simulink model "kamerol"  (R2021b)
settings: Solver=VariableStepAuto  StartTime=0.0  StopTime=10.0  RelTol=1e-3
undefined symbols (not defined in the file): admireDB
libraries: simulink_extras x104, simulink x24, sharedutil x1
(part 3 of 14)

== system kamerol/Aerodynamics/CentripetalForceCoefficient/MachRegion4/Ccday ==
  in_bus : Inport
  Bus Selector : BusSelector  OutputSignals=AeroIn_Bus.angleOfAttack_deg,AeroIn_Bus.dEY,AeroIn_Bus.mach_nd,AeroIn_Bus.qacorr,eoeff,AeroIn_Bus.dAY
  Ccday_ : Subsystem
  Ccday : Outport
  wires:
  Bus Selector/6 -> Ccday_/6(dAY)  "<dAY>"
  Bus Selector/5 -> Ccday_/5(eoeff)  "<eoeff>"
  Bus Selector/4 -> Ccday_/4(qacorr)  "<qacorr>"
  Bus Selector/3 -> Ccday_/3(mach_nd)  "<mach_nd>"
  Bus Selector/2 -> Ccday_/2(dEY)  "<dEY>"
  Bus Selector/1 -> Ccday_/1(angleOfAttack_deg)  "<angleOfAttack_deg>"
  Ccday_/1(Ccday) -> Ccday/1
  in_bus/1 -> Bus Selector/1  "in_bus"

== system kamerol/Aerodynamics/CentripetalForceCoefficient/MachRegion4/Ccdayb ==
  Constant : Constant  Value=0
  Ccdayb : Outport
  wires:
  Constant/1 -> Ccdayb/1

== system kamerol/Aerodynamics/CentripetalForceCoefficient/MachRegion4/Ccdna ==
  in_bus : Inport
  Bus Selector : BusSelector  OutputSignals=AeroIn_Bus.angleOfAttack_deg,AeroIn_Bus.mach_nd,AeroIn_Bus.dNA
  Ccdna_ : Subsystem
  Ccdna : Outport
  wires:
  Bus Selector/1 -> Ccdna_/1(angleOfAttack_deg)  "<angleOfAttack_deg>"
  Bus Selector/3 -> Ccdna_/3(dNA)  "<dNA>"
  Bus Selector/2 -> Ccdna_/2(mach_nd)  "<mach_nd>"
  in_bus/1 -> Bus Selector/1  "in_bus"
  Ccdna_/1(Ccdna) -> Ccdna/1

== system kamerol/Aerodynamics/CentripetalForceCoefficient/MachRegion4/Ccdr ==
  in_bus : Inport
  Bus Selector : BusSelector  OutputSignals=AeroIn_Bus.angleOfAttack_deg,AeroIn_Bus.mach_nd,AeroIn_Bus.rud_deg,AeroIn_Bus.qacorr
  Ccdr_ : Subsystem
  Ccdr : Outport
  wires:
  Bus Selector/1 -> Ccdr_/1(angleOfAttack_deg)  "<angleOfAttack_deg>"
  Bus Selector/2 -> Ccdr_/2(mach_nd)  "<mach_nd>"
  Bus Selector/3 -> Ccdr_/3(dR)  "<rud_deg>"
  Bus Selector/4 -> Ccdr_/4(qacorr)  "<qacorr>"
  Ccdr_/1(Ccdr) -> Ccdr/1
  in_bus/1 -> Bus Selector/1  "in_bus"

== system kamerol/Aerodynamics/CentripetalForceCoefficient/MachRegion4/Ccp ==
  in_bus : Inport
  Bus Selector : BusSelector  OutputSignals=AeroIn_Bus.angleOfAttack_deg,AeroIn_Bus.mach_nd,AeroIn_Bus.pc
  Ccp_ : Subsystem
  Ccp : Outport
  wires:
  Bus Selector/1 -> Ccp_/1(angleOfAttack_deg)  "<angleOfAttack_deg>"
  Bus Selector/2 -> Ccp_/2(mach_nd)  "<mach_nd>"
  Bus Selector/3 -> Ccp_/3(pc)  "<pc>"
  in_bus/1 -> Bus Selector/1  "in_bus"
  Ccp_/1(Ccp) -> Ccp/1

== system kamerol/Aerodynamics/CentripetalForceCoefficient/MachRegion4/Ccpbeta ==
  Constant : Constant  Value=0
  Ccpbeta : Outport
  wires:
  Constant/1 -> Ccpbeta/1

== system kamerol/Aerodynamics/CentripetalForceCoefficient/MachRegion4/Ccr ==
  in_bus : Inport
  Bus Selector : BusSelector  OutputSignals=AeroIn_Bus.mach_nd,AeroIn_Bus.qacorr,AeroIn_Bus.rc
  Ccr_ : Subsystem
  Ccr : Outport
  wires:
  Bus Selector/3 -> Ccr_/3(rc)  "<rc>"
  Bus Selector/2 -> Ccr_/2(qacorr)  "<qacorr>"
  Bus Selector/1 -> Ccr_/1(mach_nd)  "<mach_nd>"
  in_bus/1 -> Bus Selector/1  "in_bus"
  Ccr_/1(Ccr) -> Ccr/1

== system kamerol/Aerodynamics/CentripetalForceCoefficient/MachRegion4/Ccrbeta ==
  Constant : Constant  Value=0
  Ccrbeta : Outport
  wires:
  Constant/1 -> Ccrbeta/1

== system kamerol/Aerodynamics/CentripetalForceCoefficient/MachRegion4/eoeff ==
  AeroIn_Bus : Inport
  Bus Selector : BusSelector  OutputSignals=mach_nd
  CCDAYOD_M : Lookup_n-D  NumberOfTableDimensions=1  BreakpointsForDimension1=admireDB.aerodata_asym_ext.CCDAYOD.breakpoints.M  BreakpointsForDimension3=[5, 7]  Table=admireDB.aerodata_asym_ext.CCDAYOD.newTable  ExtrapMethod=Clip  InternalRulePriority=Speed  RndMeth=Simplest  InputSameDT=on
  Constant : Constant
  Sum : Sum  Inputs=-+|
  eoeff : Outport
  eieff : Outport  Port=2
  wires:
  Sum/1 -> eieff/1
  CCDAYOD_M/1 -> eoeff/1, Sum/1
  Constant/1 -> Sum/2
  Bus Selector/1 -> CCDAYOD_M/1  "<mach_nd>"
  AeroIn_Bus/1 -> Bus Selector/1

== system kamerol/Aerodynamics/NormalForceCoefficient/MachRegion1/Cnalfa ==
  in_bus : Inport
  Bus Selector : BusSelector  OutputSignals=AeroIn_Bus.angleOfAttack_deg,AeroIn_Bus.mach_nd,AeroIn_Bus.qacorr
  CNDEAL_DE_ALFA : Lookup_n-D  BreakpointsForDimension1=admireDB.aerodata_sym.CNDEAL.breakpoints.ALFA  BreakpointsForDimension2=admireDB.aerodata_sym.CNDEAL.breakpoints.DE  BreakpointsForDimension3=[5, 7]  Table=admireDB.aerodata_sym.CNDEAL.newTable  ExtrapMethod=Clip  InternalRulePriority=Speed  RndMeth=Simplest  InputSameDT=on
      settings: InputPortMap=u0,u1
  CNEA_QA_M : Lookup_n-D  BreakpointsForDimension1=admireDB.aerodata_sym.CNEA.breakpoints.M  BreakpointsForDimension2=admireDB.aerodata_sym.CNEA.breakpoints.QA  BreakpointsForDimension3=[5, 7]  Table=admireDB.aerodata_sym.CNEA.newTable  ExtrapMethod=Clip  InternalRulePriority=Speed  RndMeth=Simplest  InputSameDT=on
      settings: InputPortMap=u0,u1
  Constant : Constant  Value=0
  Product : Product
  Cnalfa : Outport
  wires:
  Product/1 -> Cnalfa/1
  CNDEAL_DE_ALFA/1 -> Product/1
  CNEA_QA_M/1 -> Product/2
  Bus Selector/2 -> CNEA_QA_M/1  "<mach_nd>"
  Bus Selector/3 -> CNEA_QA_M/2  "<qacorr>"
  Constant/1 -> CNDEAL_DE_ALFA/2
  Bus Selector/1 -> CNDEAL_DE_ALFA/1  "<angleOfAttack_deg>"
  in_bus/1 -> Bus Selector/1  "in_bus"

== system kamerol/Aerodynamics/NormalForceCoefficient/MachRegion1/Cnalfad ==
  in_bus : Inport
  Abs : Abs
  Bus Selector : BusSelector  OutputSignals=AeroIn_Bus.mach_nd,AeroIn_Bus.angleOfAttack_deg,AeroIn_Bus.alfad
  CNADAM_ALFA_M : Lookup_n-D  BreakpointsForDimension1=admireDB.aerodata_sym.CNADAM.breakpoints.M  BreakpointsForDimension2=admireDB.aerodata_sym.CNADAM.breakpoints.ALFA  BreakpointsForDimension3=[5, 7]  Table=admireDB.aerodata_sym.CNADAM.newTable  ExtrapMethod=Clip  InternalRulePriority=Speed  RndMeth=Simplest  InputSameDT=on
      settings: InputPortMap=u0,u1
  Product : Product
  Cnalfad : Outport
  wires:
  Abs/1 -> CNADAM_ALFA_M/2
  Bus Selector/1 -> CNADAM_ALFA_M/1  "<mach_nd>"
  Product/1 -> Cnalfad/1
  in_bus/1 -> Bus Selector/1  "in_bus"
  Bus Selector/2 -> Abs/1  "<angleOfAttack_deg>"
  CNADAM_ALFA_M/1 -> Product/1
  Bus Selector/3 -> Product/2  "<alfad>"

== system kamerol/Aerodynamics/NormalForceCoefficient/MachRegion1/Cnbasic ==
  in_bus : Inport
  Bus Selector : BusSelector  OutputSignals=AeroIn_Bus.mach_nd,AeroIn_Bus.qacorr
  CNEZERO_QA_M : Lookup_n-D  BreakpointsForDimension1=admireDB.aerodata_sym.CNEZERO.breakpoints.M  BreakpointsForDimension2=admireDB.aerodata_sym.CNEZERO.breakpoints.QA  BreakpointsForDimension3=[5, 7]  Table=admireDB.aerodata_sym.CNEZERO.newTable  ExtrapMethod=Clip  InternalRulePriority=Speed  RndMeth=Simplest  InputSameDT=on
      settings: InputPortMap=u0,u1
  CNZERO_M : Lookup_n-D  NumberOfTableDimensions=1  BreakpointsForDimension1=admireDB.aerodata_sym.CNZERO.breakpoints.M  BreakpointsForDimension3=[5, 7]  Table=admireDB.aerodata_sym.CNZERO.newTable  ExtrapMethod=Clip  InternalRulePriority=Speed  RndMeth=Simplest  InputSameDT=on
  Sum1 : Sum  Inputs=|++
  Cnbasic : Outport
  wires:
  CNEZERO_QA_M/1 -> Sum1/2
  CNZERO_M/1 -> Sum1/1
  Bus Selector/2 -> CNEZERO_QA_M/2  "<qacorr>"
  Bus Selector/1 -> CNZERO_M/1, CNEZERO_QA_M/1  "<mach_nd>"
  Sum1/1 -> Cnbasic/1
  in_bus/1 -> Bus Selector/1  "in_bus"

== system kamerol/Aerodynamics/NormalForceCoefficient/MachRegion1/Cnbeta ==
  in_bus : Inport
  Abs : Abs
  Bus Selector : BusSelector  OutputSignals=AeroIn_Bus.angleOfAttack_deg,AeroIn_Bus.dN,AeroIn_Bus.angleOfSideslip_deg
  CNBETA_DN_ALFA : Lookup_n-D  BreakpointsForDimension1=admireDB.aerodata_sym.CNBETA.breakpoints.ALFA  BreakpointsForDimension2=admireDB.aerodata_sym.CNBETA.breakpoints.DN  BreakpointsForDimension3=[5, 7]  Table=admireDB.aerodata_sym.CNBETA.newTable  ExtrapMethod=Clip  InternalRulePriority=Speed  RndMeth=Simplest  InputSameDT=on
      settings: InputPortMap=u0,u1
  CNKB_BETA : Lookup_n-D  NumberOfTableDimensions=1  BreakpointsForDimension1=admireDB.aerodata_sym.CNKB.breakpoints.BETA  BreakpointsForDimension3=[5, 7]  Table=admireDB.aerodata_sym.CNKB.newTable  ExtrapMethod=Clip  InternalRulePriority=Speed  RndMeth=Simplest  InputSameDT=on
  Product : Product
  Cnbeta : Outport
  wires:
  Product/1 -> Cnbeta/1
  CNBETA_DN_ALFA/1 -> Product/1
  CNKB_BETA/1 -> Product/2
  Abs/1 -> CNKB_BETA/1
  Bus Selector/3 -> Abs/1  "<angleOfSideslip_deg>"
  in_bus/1 -> Bus Selector/1  "in_bus"
  Bus Selector/2 -> CNBETA_DN_ALFA/2  "<dN>"
  Bus Selector/1 -> CNBETA_DN_ALFA/1  "<angleOfAttack_deg>"

== system kamerol/Aerodynamics/NormalForceCoefficient/MachRegion1/Cncai ==
  in_bus : Inport
  Bus Selector : BusSelector  OutputSignals=AeroIn_Bus.angleOfAttack_deg,AeroIn_Bus.cai
  CNCAI_CAI_ALFA : Lookup_n-D  BreakpointsForDimension1=admireDB.aerodata_sym.CNCAI.breakpoints.ALFA  BreakpointsForDimension2=admireDB.aerodata_sym.CNCAI.breakpoints.CAI  BreakpointsForDimension3=[5, 7]  Table=admireDB.aerodata_sym.CNCAI.newTable  ExtrapMethod=Clip  InternalRulePriority=Speed  RndMeth=Simplest  InputSameDT=on
      settings: InputPortMap=u0,u1
  Cncai : Outport
  wires:
  Bus Selector/1 -> CNCAI_CAI_ALFA/1  "<angleOfAttack_deg>"
  Bus Selector/2 -> CNCAI_CAI_ALFA/2  "<cai>"
  in_bus/1 -> Bus Selector/1  "in_bus"
  CNCAI_CAI_ALFA/1 -> Cncai/1

== system kamerol/Aerodynamics/NormalForceCoefficient/MachRegion1/Cndedn ==
  in_bus : Inport
  Bus Selector : BusSelector  OutputSignals=AeroIn_Bus.angleOfAttack_deg,AeroIn_Bus.dE,AeroIn_Bus.dN
  CNDNDE_ALFA_DE_DN : Lookup_n-D  NumberOfTableDimensions=3  BreakpointsForDimension1=admireDB.aerodata_sym.CNDNDE.breakpoints.ALFA  BreakpointsForDimension2=admireDB.aerodata_sym.CNDNDE.breakpoints.DE  BreakpointsForDimension3=admireDB.aerodata_sym.CNDNDE.breakpoints.DN  Table=admireDB.aerodata_sym.CNDNDE.newTable  ExtrapMethod=Clip  InternalRulePriority=Speed  RndMeth=Simplest  InputSameDT=on
      settings: InputPortMap=u0,u1,u2
  Cndedn : Outport
  wires:
  CNDNDE_ALFA_DE_DN/1 -> Cndedn/1
  Bus Selector/3 -> CNDNDE_ALFA_DE_DN/3  "<dN>"
  Bus Selector/2 -> CNDNDE_ALFA_DE_DN/2  "<dE>"
  Bus Selector/1 -> CNDNDE_ALFA_DE_DN/1  "<angleOfAttack_deg>"
  in_bus/1 -> Bus Selector/1  "in_bus"

== system kamerol/Aerodynamics/NormalForceCoefficient/MachRegion1/Cndei ==
  in_bus : Inport
  Bus Selector : BusSelector  OutputSignals=eieff,AeroIn_Bus.angleOfAttack_deg,AeroIn_Bus.dEI,AeroIn_Bus.mach_nd,AeroIn_Bus.qacorr
  CNDEAL_DE_ALFA : Lookup_n-D  BreakpointsForDimension1=admireDB.aerodata_sym.CNDEAL.breakpoints.ALFA  BreakpointsForDimension2=admireDB.aerodata_sym.CNDEAL.breakpoints.DE  BreakpointsForDimension3=[5, 7]  Table=admireDB.aerodata_sym.CNDEAL.newTable  ExtrapMethod=Clip  InternalRulePriority=Speed  RndMeth=Simplest  InputSameDT=on
      settings: InputPortMap=u0,u1
  CNDEAL_DE_ALFA1 : Lookup_n-D  BreakpointsForDimension1=admireDB.aerodata_sym.CNDEAL.breakpoints.ALFA  BreakpointsForDimension2=admireDB.aerodata_sym.CNDEAL.breakpoints.DE  BreakpointsForDimension3=[5, 7]  Table=admireDB.aerodata_sym.CNDEAL.newTable  ExtrapMethod=Clip  InternalRulePriority=Speed  RndMeth=Simplest  InputSameDT=on
      settings: InputPortMap=u0,u1
  CNEDEI_QA_M : Lookup_n-D  BreakpointsForDimension1=admireDB.aerodata_sym.CNEDEI.breakpoints.M  BreakpointsForDimension2=admireDB.aerodata_sym.CNEDEI.breakpoints.QA  BreakpointsForDimension3=[5, 7]  Table=admireDB.aerodata_sym.CNEDEI.newTable  ExtrapMethod=Clip  InternalRulePriority=Speed  RndMeth=Simplest  InputSameDT=on
      settings: InputPortMap=u0,u1
  Constant : Constant  Value=0
  Product : Product  Inputs=3
  Sum : Sum  Inputs=|+-
  Cndei : Outport
  wires:
  CNEDEI_QA_M/1 -> Product/3
  Sum/1 -> Product/2
  Bus Selector/1 -> Product/1  "<eieff>"
  Bus Selector/4 -> CNEDEI_QA_M/1  "<mach_nd>"
  Bus Selector/5 -> CNEDEI_QA_M/2  "<qacorr>"
  CNDEAL_DE_ALFA1/1 -> Sum/2
  Constant/1 -> CNDEAL_DE_ALFA1/2
  CNDEAL_DE_ALFA/1 -> Sum/1
  Bus Selector/2 -> CNDEAL_DE_ALFA/1, CNDEAL_DE_ALFA1/1  "<angleOfAttack_deg>"
  Bus Selector/3 -> CNDEAL_DE_ALFA/2  "<dEI>"
  in_bus/1 -> Bus Selector/1  "in_bus"
  Product/1 -> Cndei/1

== system kamerol/Aerodynamics/NormalForceCoefficient/MachRegion1/Cndey ==
  in_bus : Inport
  Bus Selector : BusSelector  OutputSignals=eoeff,AeroIn_Bus.angleOfAttack_deg,AeroIn_Bus.dEY,AeroIn_Bus.mach_nd,AeroIn_Bus.qacorr
  CNDEAL_DE_ALFA : Lookup_n-D  BreakpointsForDimension1=admireDB.aerodata_sym.CNDEAL.breakpoints.ALFA  BreakpointsForDimension2=admireDB.aerodata_sym.CNDEAL.breakpoints.DE  BreakpointsForDimension3=[5, 7]  Table=admireDB.aerodata_sym.CNDEAL.newTable  ExtrapMethod=Clip  InternalRulePriority=Speed  RndMeth=Simplest  InputSameDT=on
      settings: InputPortMap=u0,u1
  CNDEAL_DE_ALFA1 : Lookup_n-D  BreakpointsForDimension1=admireDB.aerodata_sym.CNDEAL.breakpoints.ALFA  BreakpointsForDimension2=admireDB.aerodata_sym.CNDEAL.breakpoints.DE  BreakpointsForDimension3=[5, 7]  Table=admireDB.aerodata_sym.CNDEAL.newTable  ExtrapMethod=Clip  InternalRulePriority=Speed  RndMeth=Simplest  InputSameDT=on
      settings: InputPortMap=u0,u1
  CNEDEY_QA_M : Lookup_n-D  BreakpointsForDimension1=admireDB.aerodata_sym.CNEDEY.breakpoints.M  BreakpointsForDimension2=admireDB.aerodata_sym.CNEDEY.breakpoints.QA  BreakpointsForDimension3=[5, 7]  Table=admireDB.aerodata_sym.CNEDEY.newTable  ExtrapMethod=Clip  InternalRulePriority=Speed  RndMeth=Simplest  InputSameDT=on
      settings: InputPortMap=u0,u1
  Constant : Constant  Value=0
  Product : Product  Inputs=3
  Sum : Sum  Inputs=|+-
  Cndey : Outport
  wires:
  Product/1 -> Cndey/1
  in_bus/1 -> Bus Selector/1  "in_bus"
  Bus Selector/3 -> CNDEAL_DE_ALFA/2  "<dEY>"
  Bus Selector/2 -> CNDEAL_DE_ALFA/1, CNDEAL_DE_ALFA1/1  "<angleOfAttack_deg>"
  CNDEAL_DE_ALFA/1 -> Sum/1
  Constant/1 -> CNDEAL_DE_ALFA1/2
  CNDEAL_DE_ALFA1/1 -> Sum/2
  Bus Selector/5 -> CNEDEY_QA_M/2  "<qacorr>"
  Bus Selector/4 -> CNEDEY_QA_M/1  "<mach_nd>"
  Bus Selector/1 -> Product/1  "<eoeff>"
  Sum/1 -> Product/2
  CNEDEY_QA_M/1 -> Product/3

== system kamerol/Aerodynamics/NormalForceCoefficient/MachRegion1/Cndle ==
  in_bus : Inport
  Bus Selector : BusSelector  OutputSignals=AeroIn_Bus.dN,AeroIn_Bus.angleOfAttack_deg,AeroIn_Bus.dE,AeroIn_Bus.lef_deg
  CNDLDEAL_DE_ALFA : Lookup_n-D  BreakpointsForDimension1=admireDB.aerodata_sym.CNDLDEAL.breakpoints.ALFA  BreakpointsForDimension2=admireDB.aerodata_sym.CNDLDEAL.breakpoints.DE  BreakpointsForDimension3=[5, 7]  Table=admireDB.aerodata_sym.CNDLDEAL.newTable  ExtrapMethod=Clip  InternalRulePriority=Speed  RndMeth=Simplest  InputSameDT=on
      settings: InputPortMap=u0,u1
  CNDLDNAL_DN_ALFA : Lookup_n-D  BreakpointsForDimension1=admireDB.aerodata_sym.CNDLDNAL.breakpoints.ALFA  BreakpointsForDimension2=admireDB.aerodata_sym.CNDLDNAL.breakpoints.DN  BreakpointsForDimension3=[5, 7]  Table=admireDB.aerodata_sym.CNDLDNAL.newTable  ExtrapMethod=Clip  InternalRulePriority=Speed  RndMeth=Simplest  InputSameDT=on
      settings: InputPortMap=u0,u1
  CNDLEAL_ALFA : Lookup_n-D  NumberOfTableDimensions=1  BreakpointsForDimension1=admireDB.aerodata_sym.CNDLEAL.breakpoints.ALFA  BreakpointsForDimension3=[5, 7]  Table=admireDB.aerodata_sym.CNDLEAL.newTable  ExtrapMethod=Clip  InternalRulePriority=Speed  RndMeth=Simplest  InputSameDT=on
  Constant : Constant  Value=1/27
  Product : Product  Inputs=3
  Sum : Sum  Inputs=+++
  Cndle : Outport
  wires:
  Product/1 -> Cndle/1
  Sum/1 -> Product/1
  Constant/1 -> Product/2
  Bus Selector/4 -> Product/3  "<lef_deg>"
  CNDLEAL_ALFA/1 -> Sum/2
  CNDLDNAL_DN_ALFA/1 -> Sum/1
  CNDLDEAL_DE_ALFA/1 -> Sum/3
  Bus Selector/3 -> CNDLDEAL_DE_ALFA/1  "<dE>"
  Bus Selector/2 -> CNDLEAL_ALFA/1, CNDLDNAL_DN_ALFA/1, CNDLDEAL_DE_ALFA/2  "<angleOfAttack_deg>"
  Bus Selector/1 -> CNDLDNAL_DN_ALFA/2  "<dN>"
  in_bus/1 -> Bus Selector/1  "in_bus"

== system kamerol/Aerodynamics/NormalForceCoefficient/MachRegion1/Cndn ==
  in_bus : Inport
  Bus Selector : BusSelector  OutputSignals=AeroIn_Bus.angleOfAttack_deg,AeroIn_Bus.dN,AeroIn_Bus.mach_nd,AeroIn_Bus.qacorr
  CNDNAL_DN_ALFA : Lookup_n-D  BreakpointsForDimension1=admireDB.aerodata_sym.CNDNAL.breakpoints.ALFA  BreakpointsForDimension2=admireDB.aerodata_sym.CNDNAL.breakpoints.DN  BreakpointsForDimension3=[5, 7]  Table=admireDB.aerodata_sym.CNDNAL.newTable  ExtrapMethod=Clip  InternalRulePriority=Speed  RndMeth=Simplest  InputSameDT=on
      settings: InputPortMap=u0,u1
  CNEDN_QA_M : Lookup_n-D  BreakpointsForDimension1=admireDB.aerodata_sym.CNEDN.breakpoints.M  BreakpointsForDimension2=admireDB.aerodata_sym.CNEDN.breakpoints.QA  BreakpointsForDimension3=[5, 7]  Table=admireDB.aerodata_sym.CNEDN.newTable  ExtrapMethod=Clip  InternalRulePriority=Speed  RndMeth=Simplest  InputSameDT=on
      settings: InputPortMap=u0,u1
  Product : Product
  Cndn : Outport
  wires:
  Product/1 -> Cndn/1
  CNDNAL_DN_ALFA/1 -> Product/1
  CNEDN_QA_M/1 -> Product/2
  Bus Selector/3 -> CNEDN_QA_M/1  "<mach_nd>"
  Bus Selector/4 -> CNEDN_QA_M/2  "<qacorr>"
  Bus Selector/1 -> CNDNAL_DN_ALFA/1  "<angleOfAttack_deg>"
  Bus Selector/2 -> CNDNAL_DN_ALFA/2  "<dN>"
  in_bus/1 -> Bus Selector/1  "in_bus"

== system kamerol/Aerodynamics/NormalForceCoefficient/MachRegion1/Cnhigh ==
  in_bus : Inport
  Bus Selector : BusSelector  OutputSignals=AeroIn_Bus.angleOfAttack_deg,AeroIn_Bus.dN,AeroIn_Bus.dE
  CNHDE_DE_ALFA : Lookup_n-D  BreakpointsForDimension1=admireDB.aerodata_high.CNHDE.breakpoints.ALFA  BreakpointsForDimension2=admireDB.aerodata_high.CNHDE.breakpoints.DE  BreakpointsForDimension3=[5, 7]  Table=admireDB.aerodata_high.CNHDE.newTable  ExtrapMethod=Clip  InternalRulePriority=Speed  RndMeth=Simplest  InputSameDT=on
      settings: InputPortMap=u0,u1
  CNHDN_DN_ALFA : Lookup_n-D  BreakpointsForDimension1=admireDB.aerodata_high.CNHDN.breakpoints.ALFA  BreakpointsForDimension2=admireDB.aerodata_high.CNHDN.breakpoints.DN  BreakpointsForDimension3=[5, 7]  Table=admireDB.aerodata_high.CNHDN.newTable  ExtrapMethod=Clip  InternalRulePriority=Speed  RndMeth=Simplest  InputSameDT=on
      settings: InputPortMap=u0,u1
  CNHZERO_ALFA : Lookup_n-D  NumberOfTableDimensions=1  BreakpointsForDimension1=admireDB.aerodata_high.CNHZERO.breakpoints.ALFA  BreakpointsForDimension3=[5, 7]  Table=admireDB.aerodata_high.CNHZERO.newTable  ExtrapMethod=Clip  InternalRulePriority=Speed  RndMeth=Simplest  InputSameDT=on
  Sum : Sum  Inputs=+++
  Cnhigh : Outport
  wires:
  CNHZERO_ALFA/1 -> Sum/1
  CNHDE_DE_ALFA/1 -> Sum/3
  CNHDN_DN_ALFA/1 -> Sum/2
  Bus Selector/3 -> CNHDE_DE_ALFA/2  "<dE>"
  Bus Selector/2 -> CNHDN_DN_ALFA/2  "<dN>"
  Bus Selector/1 -> CNHZERO_ALFA/1, CNHDN_DN_ALFA/1, CNHDE_DE_ALFA/1  "<angleOfAttack_deg>"
  Sum/1 -> Cnhigh/1
  in_bus/1 -> Bus Selector/1  "in_bus"

== system kamerol/Aerodynamics/NormalForceCoefficient/MachRegion1/Cnlg ==
  in_bus : Inport
  Abs : Abs
  Bus Selector : BusSelector  OutputSignals=AeroIn_Bus.angleOfAttack_deg,AeroIn_Bus.angleOfSideslip_deg,AeroIn_Bus.lg_bool
  CNLST_BETA_ALFA : Lookup_n-D  BreakpointsForDimension1=admireDB.aerodata_sym.CNLST.breakpoints.ALFA  BreakpointsForDimension2=admireDB.aerodata_sym.CNLST.breakpoints.BETA  BreakpointsForDimension3=[5, 7]  Table=admireDB.aerodata_sym.CNLST.newTable  ExtrapMethod=Clip  InternalRulePriority=Speed  RndMeth=Simplest  InputSameDT=on
      settings: InputPortMap=u0,u1
  Product : Product
  Cnlg : Outport
  wires:
  Bus Selector/3 -> Product/2  "<lg_bool>"
  CNLST_BETA_ALFA/1 -> Product/1
  Abs/1 -> CNLST_BETA_ALFA/2
  Bus Selector/1 -> CNLST_BETA_ALFA/1  "<angleOfAttack_deg>"
  Bus Selector/2 -> Abs/1  "<angleOfSideslip_deg>"
  in_bus/1 -> Bus Selector/1  "in_bus"
  Product/1 -> Cnlg/1

== system kamerol/Aerodynamics/NormalForceCoefficient/MachRegion1/Cnnz ==
  in_bus : Inport
  Bus Selector : BusSelector  OutputSignals=AeroIn_Bus.nz_g,AeroIn_Bus.mach_nd,AeroIn_Bus.qacorr
  CNENZ_QA_M : Lookup_n-D  BreakpointsForDimension1=admireDB.aerodata_sym.CNENZ.breakpoints.M  BreakpointsForDimension2=admireDB.aerodata_sym.CNENZ.breakpoints.QA  BreakpointsForDimension3=[5, 7]  Table=admireDB.aerodata_sym.CNENZ.newTable  ExtrapMethod=Clip  InternalRulePriority=Speed  RndMeth=Simplest  InputSameDT=on
      settings: InputPortMap=u0,u1
  Constant : Constant
  Product : Product
  Sum : Sum  Inputs=-+|
  Cnnz : Outport
  wires:
  CNENZ_QA_M/1 -> Product/2
  Sum/1 -> Product/1
  Constant/1 -> Sum/1
  Product/1 -> Cnnz/1
  in_bus/1 -> Bus Selector/1  "in_bus"
  Bus Selector/1 -> Sum/2  "<nz_g>"
  Bus Selector/3 -> CNENZ_QA_M/2  "<qacorr>"
  Bus Selector/2 -> CNENZ_QA_M/1  "<mach_nd>"

== system kamerol/Aerodynamics/NormalForceCoefficient/MachRegion1/Cnq ==
  in_bus : Inport
  Abs : Abs
  Bus Selector : BusSelector  OutputSignals=AeroIn_Bus.angleOfAttack_deg,AeroIn_Bus.qc,AeroIn_Bus.mach_nd,AeroIn_Bus.qacorr
  CNEQ_QA_M : Lookup_n-D  BreakpointsForDimension1=admireDB.aerodata_sym.CNEQ.breakpoints.M  BreakpointsForDimension2=admireDB.aerodata_sym.CNEQ.breakpoints.QA  BreakpointsForDimension3=[5, 7]  Table=admireDB.aerodata_sym.CNEQ.newTable  ExtrapMethod=Clip  InternalRulePriority=Speed  RndMeth=Simplest  InputSameDT=on
      settings: InputPortMap=u0,u1
  CNQAL_ALFA : Lookup_n-D  NumberOfTableDimensions=1  BreakpointsForDimension1=admireDB.aerodata_sym.CNQAL.breakpoints.ALFA  BreakpointsForDimension3=[5, 7]  Table=admireDB.aerodata_sym.CNQAL.newTable  ExtrapMethod=Clip  InternalRulePriority=Speed  RndMeth=Simplest  InputSameDT=on
  Product : Product  Inputs=3
  Cnq : Outport
  wires:
  Bus Selector/2 -> Product/2  "<qc>"
  CNQAL_ALFA/1 -> Product/1
  CNEQ_QA_M/1 -> Product/3
  Bus Selector/3 -> CNEQ_QA_M/1  "<mach_nd>"
  Bus Selector/4 -> CNEQ_QA_M/2  "<qacorr>"
  Abs/1 -> CNQAL_ALFA/1
  Bus Selector/1 -> Abs/1  "<angleOfAttack_deg>"
  in_bus/1 -> Bus Selector/1  "in_bus"
  Product/1 -> Cnq/1

== system kamerol/Aerodynamics/NormalForceCoefficient/MachRegion1/Cnqd ==
  in_bus : Inport
  Bus Selector : BusSelector  OutputSignals=AeroIn_Bus.qd,AeroIn_Bus.mach_nd,AeroIn_Bus.qacorr
  CNEQD_QA_M : Lookup_n-D  BreakpointsForDimension1=admireDB.aerodata_sym.CNEQD.breakpoints.M  BreakpointsForDimension2=admireDB.aerodata_sym.CNEQD.breakpoints.QA  BreakpointsForDimension3=[5, 7]  Table=admireDB.aerodata_sym.CNEQD.newTable  ExtrapMethod=Clip  InternalRulePriority=Speed  RndMeth=Simplest  InputSameDT=on
      settings: InputPortMap=u0,u1
  Product : Product
  Cnqd : Outport
  wires:
  Bus Selector/2 -> CNEQD_QA_M/1  "<mach_nd>"
  Bus Selector/3 -> CNEQD_QA_M/2  "<qacorr>"
  Bus Selector/1 -> Product/1  "<qd>"
  in_bus/1 -> Bus Selector/1  "in_bus"
  Product/1 -> Cnqd/1
  CNEQD_QA_M/1 -> Product/2

== system kamerol/Aerodynamics/NormalForceCoefficient/MachRegion1/eoeff ==
  AeroIn_Bus : Inport
  Abs : Abs
  Bus Selector : BusSelector  OutputSignals=mach_nd,angleOfAttack_deg
  CNDEYODE_ALFA_M : Lookup_n-D  BreakpointsForDimension1=admireDB.aerodata_sym.CNDEYODE.breakpoints.M  BreakpointsForDimension2=admireDB.aerodata_sym.CNDEYODE.breakpoints.ALFA  BreakpointsForDimension3=[5, 7]  Table=admireDB.aerodata_sym.CNDEYODE.newTable  ExtrapMethod=Clip  InternalRulePriority=Speed  RndMeth=Simplest  InputSameDT=on
      settings: InputPortMap=u0,u1
  Constant : Constant
  Sum : Sum  Inputs=-+|
  eoeff : Outport
  eieff : Outport  Port=2
  wires:
  Abs/1 -> CNDEYODE_ALFA_M/2
  Bus Selector/2 -> Abs/1  "<angleOfAttack_deg>"
  Sum/1 -> eieff/1
  CNDEYODE_ALFA_M/1 -> eoeff/1, Sum/1
  Constant/1 -> Sum/2
  Bus Selector/1 -> CNDEYODE_ALFA_M/1  "<mach_nd>"
  AeroIn_Bus/1 -> Bus Selector/1

== system kamerol/Aerodynamics/NormalForceCoefficient/MachRegion2/Cnalfa ==
  in_bus : Inport
  Bus Selector : BusSelector  OutputSignals=AeroIn_Bus.angleOfAttack_deg,AeroIn_Bus.tflow,AeroIn_Bus.tfhigh,AeroIn_Bus.mach_nd,AeroIn_Bus.qacorr
  CNDEAL_DE_ALFA : Lookup_n-D  BreakpointsForDimension1=admireDB.aerodata_sym.CNDEAL.breakpoints.ALFA  BreakpointsForDimension2=admireDB.aerodata_sym.CNDEAL.breakpoints.DE  BreakpointsForDimension3=[5, 7]  Table=admireDB.aerodata_sym.CNDEAL.newTable  ExtrapMethod=Clip  InternalRulePriority=Speed  RndMeth=Simplest  InputSameDT=on
      settings: InputPortMap=u0,u1
  CNEA_QA_M : Lookup_n-D  BreakpointsForDimension1=admireDB.aerodata_sym.CNEA.breakpoints.M  BreakpointsForDimension2=admireDB.aerodata_sym.CNEA.breakpoints.QA  BreakpointsForDimension3=[5, 7]  Table=admireDB.aerodata_sym.CNEA.newTable  ExtrapMethod=Clip  InternalRulePriority=Speed  RndMeth=Simplest  InputSameDT=on
      settings: InputPortMap=u0,u1
  CNMDEA_ALFA_DE_M : Lookup_n-D  NumberOfTableDimensions=3  BreakpointsForDimension1=admireDB.aerodata_sym.CNMDEA.breakpoints.ALFA  BreakpointsForDimension2=admireDB.aerodata_sym.CNMDEA.breakpoints.DE  BreakpointsForDimension3=admireDB.aerodata_sym.CNMDEA.breakpoints.M  Table=admireDB.aerodata_sym.CNMDEA.newTable  ExtrapMethod=Clip  InternalRulePriority=Speed  RndMeth=Simplest  InputSameDT=on
      settings: InputPortMap=u0,u1,u2
  Constant : Constant  Value=0
  Product : Product
  Product1 : Product
  Product2 : Product
  Sum : Sum  Inputs=++|
  dE_cnst : Constant  Value=0.0
  mach_nd_cnst : Constant  Value=0.5
  Cnalfa : Outport
  wires:
  Product2/1 -> Cnalfa/1
  Sum/1 -> Product2/1
  Product1/1 -> Sum/2
  CNEA_QA_M/1 -> Product2/2
  Bus Selector/4 -> CNEA_QA_M/1  "<mach_nd>"
  Bus Selector/5 -> CNEA_QA_M/2  "<qacorr>"
  Bus Selector/3 -> Product1/1  "<tfhigh>"
  CNMDEA_ALFA_DE_M/1 -> Product1/2
  mach_nd_cnst/1 -> CNMDEA_ALFA_DE_M/3
  dE_cnst/1 -> CNMDEA_ALFA_DE_M/2
  Bus Selector/2 -> Product/2  "<tflow>"
  in_bus/1 -> Bus Selector/1  "in_bus"
  Bus Selector/1 -> CNMDEA_ALFA_DE_M/1, CNDEAL_DE_ALFA/1  "<angleOfAttack_deg>"
  Constant/1 -> CNDEAL_DE_ALFA/2
  CNDEAL_DE_ALFA/1 -> Product/1
  Product/1 -> Sum/1

== system kamerol/Aerodynamics/NormalForceCoefficient/MachRegion2/Cnalfad ==
  in_bus : Inport
  Abs : Abs
  Bus Selector : BusSelector  OutputSignals=AeroIn_Bus.mach_nd,AeroIn_Bus.angleOfAttack_deg,AeroIn_Bus.alfad
  CNADAM_ALFA_M : Lookup_n-D  BreakpointsForDimension1=admireDB.aerodata_sym.CNADAM.breakpoints.M  BreakpointsForDimension2=admireDB.aerodata_sym.CNADAM.breakpoints.ALFA  BreakpointsForDimension3=[5, 7]  Table=admireDB.aerodata_sym.CNADAM.newTable  ExtrapMethod=Clip  InternalRulePriority=Speed  RndMeth=Simplest  InputSameDT=on
      settings: InputPortMap=u0,u1
  Product : Product
  Cnalfad : Outport
  wires:
  Bus Selector/3 -> Product/2  "<alfad>"
  CNADAM_ALFA_M/1 -> Product/1
  Bus Selector/2 -> Abs/1  "<angleOfAttack_deg>"
  in_bus/1 -> Bus Selector/1  "in_bus"
  Product/1 -> Cnalfad/1
  Bus Selector/1 -> CNADAM_ALFA_M/1  "<mach_nd>"
  Abs/1 -> CNADAM_ALFA_M/2

== system kamerol/Aerodynamics/NormalForceCoefficient/MachRegion2/Cnbasic ==
  in_bus : Inport
  Bus Selector : BusSelector  OutputSignals=AeroIn_Bus.mach_nd,AeroIn_Bus.qacorr
  CNEZERO_QA_M : Lookup_n-D  BreakpointsForDimension1=admireDB.aerodata_sym.CNEZERO.breakpoints.M  BreakpointsForDimension2=admireDB.aerodata_sym.CNEZERO.breakpoints.QA  BreakpointsForDimension3=[5, 7]  Table=admireDB.aerodata_sym.CNEZERO.newTable  ExtrapMethod=Clip  InternalRulePriority=Speed  RndMeth=Simplest  InputSameDT=on
      settings: InputPortMap=u0,u1
  CNZERO_M : Lookup_n-D  NumberOfTableDimensions=1  BreakpointsForDimension1=admireDB.aerodata_sym.CNZERO.breakpoints.M  BreakpointsForDimension3=[5, 7]  Table=admireDB.aerodata_sym.CNZERO.newTable  ExtrapMethod=Clip  InternalRulePriority=Speed  RndMeth=Simplest  InputSameDT=on
  Sum1 : Sum  Inputs=|++
  Cnbasic : Outport
  wires:
  in_bus/1 -> Bus Selector/1  "in_bus"
  Sum1/1 -> Cnbasic/1
  Bus Selector/1 -> CNZERO_M/1, CNEZERO_QA_M/1  "<mach_nd>"
  Bus Selector/2 -> CNEZERO_QA_M/2  "<qacorr>"
  CNZERO_M/1 -> Sum1/1
  CNEZERO_QA_M/1 -> Sum1/2

== system kamerol/Aerodynamics/NormalForceCoefficient/MachRegion2/Cnbeta ==
  in_bus : Inport
  Abs : Abs
  Bus Selector : BusSelector  OutputSignals=AeroIn_Bus.angleOfAttack_deg,AeroIn_Bus.dN,AeroIn_Bus.angleOfSideslip_deg,AeroIn_Bus.tflow
  CNBETA_DN_ALFA : Lookup_n-D  BreakpointsForDimension1=admireDB.aerodata_sym.CNBETA.breakpoints.ALFA  BreakpointsForDimension2=admireDB.aerodata_sym.CNBETA.breakpoints.DN  BreakpointsForDimension3=[5, 7]  Table=admireDB.aerodata_sym.CNBETA.newTable  ExtrapMethod=Clip  InternalRulePriority=Speed  RndMeth=Simplest  InputSameDT=on
      settings: InputPortMap=u0,u1
  CNKB_BETA : Lookup_n-D  NumberOfTableDimensions=1  BreakpointsForDimension1=admireDB.aerodata_sym.CNKB.breakpoints.BETA  BreakpointsForDimension3=[5, 7]  Table=admireDB.aerodata_sym.CNKB.newTable  ExtrapMethod=Clip  InternalRulePriority=Speed  RndMeth=Simplest  InputSameDT=on
  Product : Product  Inputs=3
  Cnbeta : Outport
  wires:
  Bus Selector/4 -> Product/3  "<tflow>"
  Bus Selector/1 -> CNBETA_DN_ALFA/1  "<angleOfAttack_deg>"
  Bus Selector/2 -> CNBETA_DN_ALFA/2  "<dN>"
  in_bus/1 -> Bus Selector/1  "in_bus"
  Bus Selector/3 -> Abs/1  "<angleOfSideslip_deg>"
  Abs/1 -> CNKB_BETA/1
  CNKB_BETA/1 -> Product/2
  CNBETA_DN_ALFA/1 -> Product/1
  Product/1 -> Cnbeta/1

== system kamerol/Aerodynamics/NormalForceCoefficient/MachRegion2/Cncai ==
  in_bus : Inport
  Bus Selector : BusSelector  OutputSignals=AeroIn_Bus.angleOfAttack_deg,AeroIn_Bus.cai
  CNCAI_CAI_ALFA : Lookup_n-D  BreakpointsForDimension1=admireDB.aerodata_sym.CNCAI.breakpoints.ALFA  BreakpointsForDimension2=admireDB.aerodata_sym.CNCAI.breakpoints.CAI  BreakpointsForDimension3=[5, 7]  Table=admireDB.aerodata_sym.CNCAI.newTable  ExtrapMethod=Clip  InternalRulePriority=Speed  RndMeth=Simplest  InputSameDT=on
      settings: InputPortMap=u0,u1
  Cncai : Outport
  wires:
  CNCAI_CAI_ALFA/1 -> Cncai/1
  in_bus/1 -> Bus Selector/1  "in_bus"
  Bus Selector/2 -> CNCAI_CAI_ALFA/2  "<cai>"
  Bus Selector/1 -> CNCAI_CAI_ALFA/1  "<angleOfAttack_deg>"

== system kamerol/Aerodynamics/NormalForceCoefficient/MachRegion2/Cndedn ==
  in_bus : Inport
  Bus Selector : BusSelector  OutputSignals=AeroIn_Bus.angleOfAttack_deg,AeroIn_Bus.dE,AeroIn_Bus.dN,AeroIn_Bus.tflow
  CNDNDE_ALFA_DE_DN : Lookup_n-D  NumberOfTableDimensions=3  BreakpointsForDimension1=admireDB.aerodata_sym.CNDNDE.breakpoints.ALFA  BreakpointsForDimension2=admireDB.aerodata_sym.CNDNDE.breakpoints.DE  BreakpointsForDimension3=admireDB.aerodata_sym.CNDNDE.breakpoints.DN  Table=admireDB.aerodata_sym.CNDNDE.newTable  ExtrapMethod=Clip  InternalRulePriority=Speed  RndMeth=Simplest  InputSameDT=on
      settings: InputPortMap=u0,u1,u2
  Product : Product
  Cndedn : Outport
  wires:
  Bus Selector/4 -> Product/2  "<tflow>"
  CNDNDE_ALFA_DE_DN/1 -> Product/1
  Product/1 -> Cndedn/1
  in_bus/1 -> Bus Selector/1  "in_bus"
  Bus Selector/1 -> CNDNDE_ALFA_DE_DN/1  "<angleOfAttack_deg>"
  Bus Selector/2 -> CNDNDE_ALFA_DE_DN/2  "<dE>"
  Bus Selector/3 -> CNDNDE_ALFA_DE_DN/3  "<dN>"

== system kamerol/Aerodynamics/NormalForceCoefficient/MachRegion2/Cndei ==
  in_bus : Inport
  Bus Selector : BusSelector  OutputSignals=AeroIn_Bus.tflow,AeroIn_Bus.dEI,AeroIn_Bus.angleOfAttack_deg,AeroIn_Bus.dEI,AeroIn_Bus.tfhigh,eieff,AeroIn_Bus.mach_nd,AeroIn_Bus.qacorr
  CNEDEI_QA_M : Lookup_n-D  BreakpointsForDimension1=admireDB.aerodata_sym.CNEDEI.breakpoints.M  BreakpointsForDimension2=admireDB.aerodata_sym.CNEDEI.breakpoints.QA  BreakpointsForDimension3=[5, 7]  Table=admireDB.aerodata_sym.CNEDEI.newTable  ExtrapMethod=Clip  InternalRulePriority=Speed  RndMeth=Simplest  InputSameDT=on
      settings: InputPortMap=u0,u1
  Product : Product
  Product1 : Product
  Product2 : Product  Inputs=3
  Subsystem : Subsystem
  Subsystem1 : Subsystem
  Sum2 : Sum  Inputs=++|
  Cndei : Outport
  wires:
  Product2/1 -> Cndei/1
  Product/1 -> Sum2/1
  Product1/1 -> Sum2/2
  Subsystem1/1(Out1) -> Product/2
  Bus Selector/2 -> Subsystem1/1(<dEI>)  "<dEI>"
  Subsystem/1(Out1) -> Product1/1
  Bus Selector/4 -> Subsystem/1(<dEI>)  "<dEI>"
  CNEDEI_QA_M/1 -> Product2/3
  Sum2/1 -> Product2/1
  Bus Selector/6 -> Product2/2  "<eieff>"
  Bus Selector/7 -> CNEDEI_QA_M/1  "<mach_nd>"
  Bus Selector/8 -> CNEDEI_QA_M/2  "<qacorr>"
  Bus Selector/5 -> Product1/2  "<tfhigh>"
  in_bus/1 -> Bus Selector/1  "in_bus"
  Bus Selector/3 -> Subsystem/2(<angleOfAttack_deg>), Subsystem1/2(<angleOfAttack_deg>)  "<angleOfAttack_deg>"
  Bus Selector/1 -> Product/1  "<tflow>"

== system kamerol/Aerodynamics/NormalForceCoefficient/MachRegion2/Cndey ==
  in_bus : Inport
  Bus Selector : BusSelector  OutputSignals=AeroIn_Bus.tflow,AeroIn_Bus.dEY,AeroIn_Bus.angleOfAttack_deg,AeroIn_Bus.tfhigh,eoeff,AeroIn_Bus.mach_nd,AeroIn_Bus.qacorr
  CNEDEY_QA_M : Lookup_n-D  BreakpointsForDimension1=admireDB.aerodata_sym.CNEDEY.breakpoints.M  BreakpointsForDimension2=admireDB.aerodata_sym.CNEDEY.breakpoints.QA  BreakpointsForDimension3=[5, 7]  Table=admireDB.aerodata_sym.CNEDEY.newTable  ExtrapMethod=Clip  InternalRulePriority=Speed  RndMeth=Simplest  InputSameDT=on
      settings: InputPortMap=u0,u1
  Product : Product
  Product1 : Product
  Product2 : Product  Inputs=3
  Subsystem : Subsystem
  Subsystem1 : Subsystem
  Sum2 : Sum  Inputs=++|
  Cndey : Outport
  wires:
  [eoeff] -> Product2/2
  Bus Selector/1 -> Product/1  "<tflow>"
  Bus Selector/3 -> Subsystem/2(<angleOfAttack_deg>), Subsystem1/2(<angleOfAttack_deg>)  "<angleOfAttack_deg>"
  in_bus/1 -> Bus Selector/1  "in_bus"
  Bus Selector/4 -> Product1/1  "<tfhigh>"
  Bus Selector/7 -> CNEDEY_QA_M/2  "<qacorr>"
  Bus Selector/6 -> CNEDEY_QA_M/1  "<mach_nd>"
  Bus Selector/5 -> [eoeff]  "<eoeff>"
  Sum2/1 -> Product2/1
  CNEDEY_QA_M/1 -> Product2/3
  Subsystem/1(Out1) -> Product1/2
  Bus Selector/2 -> Subsystem1/1(dEY), Subsystem/1(dEY)  "<dEY>"
  Subsystem1/1(Out1) -> Product/2
  Product1/1 -> Sum2/2
  Product/1 -> Sum2/1
  Product2/1 -> Cndey/1

== system kamerol/Aerodynamics/NormalForceCoefficient/MachRegion2/Cndle ==
  in_bus : Inport
  Bus Selector : BusSelector  OutputSignals=AeroIn_Bus.dN,AeroIn_Bus.angleOfAttack_deg,AeroIn_Bus.dE,AeroIn_Bus.lef_deg,AeroIn_Bus.tflow,AeroIn_Bus.tfhigh
  CNDLDEAL_DE_ALFA : Lookup_n-D  BreakpointsForDimension1=admireDB.aerodata_sym.CNDLDEAL.breakpoints.ALFA  BreakpointsForDimension2=admireDB.aerodata_sym.CNDLDEAL.breakpoints.DE  BreakpointsForDimension3=[5, 7]  Table=admireDB.aerodata_sym.CNDLDEAL.newTable  ExtrapMethod=Clip  InternalRulePriority=Speed  RndMeth=Simplest  InputSameDT=on
      settings: InputPortMap=u0,u1
  CNDLDNAL_DN_ALFA : Lookup_n-D  BreakpointsForDimension1=admireDB.aerodata_sym.CNDLDNAL.breakpoints.ALFA  BreakpointsForDimension2=admireDB.aerodata_sym.CNDLDNAL.breakpoints.DN  BreakpointsForDimension3=[5, 7]  Table=admireDB.aerodata_sym.CNDLDNAL.newTable  ExtrapMethod=Clip  InternalRulePriority=Speed  RndMeth=Simplest  InputSameDT=on
      settings: InputPortMap=u0,u1
  CNDLEAL_ALFA : Lookup_n-D  NumberOfTableDimensions=1  BreakpointsForDimension1=admireDB.aerodata_sym.CNDLEAL.breakpoints.ALFA  BreakpointsForDimension3=[5, 7]  Table=admireDB.aerodata_sym.CNDLEAL.newTable  ExtrapMethod=Clip  InternalRulePriority=Speed  RndMeth=Simplest  InputSameDT=on
  CNMDLEA_ALFA_DLE_M : Lookup_n-D  NumberOfTableDimensions=3  BreakpointsForDimension1=admireDB.aerodata_sym.CNMDLEA.breakpoints.ALFA  BreakpointsForDimension2=admireDB.aerodata_sym.CNMDLEA.breakpoints.DLE  BreakpointsForDimension3=admireDB.aerodata_sym.CNMDLEA.breakpoints.M  Table=admireDB.aerodata_sym.CNMDLEA.newTable  ExtrapMethod=Clip  InternalRulePriority=Speed  RndMeth=Simplest  InputSameDT=on
      settings: InputPortMap=u0,u1,u2
  Constant : Constant  Value=1/27
  Product : Product  Inputs=4
  Product1 : Product
  Sum : Sum  Inputs=+++
  Sum1 : Sum  Inputs=|++
  mach_nd_cnst : Constant  Value=0.5
  Cndle : Outport
  wires:
  Product1/1 -> Sum1/2
  Sum1/1 -> Cndle/1
  Product/1 -> Sum1/1
  Bus Selector/6 -> Product1/2  "<tfhigh>"
  CNMDLEA_ALFA_DLE_M/1 -> Product1/1
  Bus Selector/5 -> Product/4  "<tflow>"
  mach_nd_cnst/1 -> CNMDLEA_ALFA_DLE_M/3
  in_bus/1 -> Bus Selector/1  "in_bus"
  Bus Selector/1 -> CNDLDNAL_DN_ALFA/2  "<dN>"
  Bus Selector/2 -> CNMDLEA_ALFA_DLE_M/1, CNDLDEAL_DE_ALFA/2, CNDLEAL_ALFA/1, CNDLDNAL_DN_ALFA/1  "<angleOfAttack_deg>"
  Bus Selector/3 -> CNDLDEAL_DE_ALFA/1  "<dE>"
  CNDLDEAL_DE_ALFA/1 -> Sum/3
  CNDLDNAL_DN_ALFA/1 -> Sum/1
  CNDLEAL_ALFA/1 -> Sum/2
  Bus Selector/4 -> Product/3, CNMDLEA_ALFA_DLE_M/2  "<lef_deg>"
  Constant/1 -> Product/2
  Sum/1 -> Product/1

== system kamerol/Aerodynamics/NormalForceCoefficient/MachRegion2/Cndn ==
  in_bus : Inport
  Bus Selector : BusSelector  OutputSignals=AeroIn_Bus.dN,AeroIn_Bus.angleOfAttack_deg,AeroIn_Bus.tflow,AeroIn_Bus.tfhigh,AeroIn_Bus.mach_nd,AeroIn_Bus.qacorr
  CNEDN_QA_M : Lookup_n-D  BreakpointsForDimension1=admireDB.aerodata_sym.CNEDN.breakpoints.M  BreakpointsForDimension2=admireDB.aerodata_sym.CNEDN.breakpoints.QA  BreakpointsForDimension3=[5, 7]  Table=admireDB.aerodata_sym.CNEDN.newTable  ExtrapMethod=Clip  InternalRulePriority=Speed  RndMeth=Simplest  InputSameDT=on
      settings: InputPortMap=u0,u1
  Product : Product
  Subsystem : Subsystem
  Subsystem1 : Subsystem
  Sum : Sum  Inputs=++|
  Cndn : Outport
  wires:
  Sum/1 -> Product/1
  Subsystem/1(Out1) -> Sum/1
  Subsystem1/1(Out1) -> Sum/2
  Bus Selector/4 -> Subsystem1/3(<tfhigh>)  "<tfhigh>"
  Bus Selector/3 -> Subsystem/3(tflow)  "<tflow>"
  Bus Selector/2 -> Subsystem/2(angleOfAttack_deg), Subsystem1/2(<angleOfAttack_deg>)  "<angleOfAttack_deg>"
  Bus Selector/1 -> Subsystem/1(dN), Subsystem1/1(<dN>)  "<dN>"
  in_bus/1 -> Bus Selector/1  "in_bus"
  Bus Selector/6 -> CNEDN_QA_M/2  "<qacorr>"
  Bus Selector/5 -> CNEDN_QA_M/1  "<mach_nd>"
  CNEDN_QA_M/1 -> Product/2
  Product/1 -> Cndn/1

== system kamerol/Aerodynamics/NormalForceCoefficient/MachRegion2/Cnhigh ==
  Constant : Constant  Value=0
  Cnhigh : Outport
  wires:
  Constant/1 -> Cnhigh/1

== system kamerol/Aerodynamics/NormalForceCoefficient/MachRegion2/Cnlg ==
  in_bus : Inport
  Abs : Abs
  Bus Selector : BusSelector  OutputSignals=AeroIn_Bus.angleOfAttack_deg,AeroIn_Bus.angleOfSideslip_deg,AeroIn_Bus.lg_bool
  CNLST_BETA_ALFA : Lookup_n-D  BreakpointsForDimension1=admireDB.aerodata_sym.CNLST.breakpoints.ALFA  BreakpointsForDimension2=admireDB.aerodata_sym.CNLST.breakpoints.BETA  BreakpointsForDimension3=[5, 7]  Table=admireDB.aerodata_sym.CNLST.newTable  ExtrapMethod=Clip  InternalRulePriority=Speed  RndMeth=Simplest  InputSameDT=on
      settings: InputPortMap=u0,u1
  Product : Product
  Cnlg : Outport
  wires:
  Product/1 -> Cnlg/1
  in_bus/1 -> Bus Selector/1  "in_bus"
  Bus Selector/2 -> Abs/1  "<angleOfSideslip_deg>"
  Bus Selector/1 -> CNLST_BETA_ALFA/1  "<angleOfAttack_deg>"
  Abs/1 -> CNLST_BETA_ALFA/2
  CNLST_BETA_ALFA/1 -> Product/1
  Bus Selector/3 -> Product/2  "<lg_bool>"

== system kamerol/Aerodynamics/NormalForceCoefficient/MachRegion2/Cnnz ==
  in_bus : Inport
  Bus Selector : BusSelector  OutputSignals=AeroIn_Bus.nz_g,AeroIn_Bus.mach_nd,AeroIn_Bus.qacorr
  CNENZ_QA_M : Lookup_n-D  BreakpointsForDimension1=admireDB.aerodata_sym.CNENZ.breakpoints.M  BreakpointsForDimension2=admireDB.aerodata_sym.CNENZ.breakpoints.QA  BreakpointsForDimension3=[5, 7]  Table=admireDB.aerodata_sym.CNENZ.newTable  ExtrapMethod=Clip  InternalRulePriority=Speed  RndMeth=Simplest  InputSameDT=on
      settings: InputPortMap=u0,u1
  Constant : Constant
  Product : Product
  Sum : Sum  Inputs=-+|
  Cnnz : Outport
  wires:
  Bus Selector/2 -> CNENZ_QA_M/1  "<mach_nd>"
  Bus Selector/3 -> CNENZ_QA_M/2  "<qacorr>"
  Bus Selector/1 -> Sum/2  "<nz_g>"
  in_bus/1 -> Bus Selector/1  "in_bus"
  Product/1 -> Cnnz/1
  Constant/1 -> Sum/1
  Sum/1 -> Product/1
  CNENZ_QA_M/1 -> Product/2

== system kamerol/Aerodynamics/NormalForceCoefficient/MachRegion2/Cnq ==
  in_bus : Inport
  Bus Selector : BusSelector  OutputSignals=AeroIn_Bus.angleOfAttack_deg,AeroIn_Bus.tflow,AeroIn_Bus.tfhigh,AeroIn_Bus.qc,AeroIn_Bus.mach_nd,AeroIn_Bus.qacorr
  CNEQ_QA_M : Lookup_n-D  BreakpointsForDimension1=admireDB.aerodata_sym.CNEQ.breakpoints.M  BreakpointsForDimension2=admireDB.aerodata_sym.CNEQ.breakpoints.QA  BreakpointsForDimension3=[5, 7]  Table=admireDB.aerodata_sym.CNEQ.newTable  ExtrapMethod=Clip  InternalRulePriority=Speed  RndMeth=Simplest  InputSameDT=on
      settings: InputPortMap=u0,u1
  Product : Product  Inputs=3
  Subsystem : Subsystem
  Cnq : Outport
  wires:
  Bus Selector/4 -> Product/2  "<qc>"
  CNEQ_QA_M/1 -> Product/3
  Subsystem/1(Out1) -> Product/1
  Bus Selector/3 -> Subsystem/3(<tfhigh>)  "<tfhigh>"
  Bus Selector/2 -> Subsystem/2(<tflow>)  "<tflow>"
  Bus Selector/1 -> Subsystem/1(<angleOfAttack_deg>)  "<angleOfAttack_deg>"
  Product/1 -> Cnq/1
  in_bus/1 -> Bus Selector/1  "in_bus"
  Bus Selector/6 -> CNEQ_QA_M/2  "<qacorr>"
  Bus Selector/5 -> CNEQ_QA_M/1  "<mach_nd>"

== system kamerol/Aerodynamics/NormalForceCoefficient/MachRegion2/Cnqd ==
  in_bus : Inport
  Bus Selector : BusSelector  OutputSignals=AeroIn_Bus.qd,AeroIn_Bus.mach_nd,AeroIn_Bus.qacorr
  CNEQD_QA_M : Lookup_n-D  BreakpointsForDimension1=admireDB.aerodata_sym.CNEQD.breakpoints.M  BreakpointsForDimension2=admireDB.aerodata_sym.CNEQD.breakpoints.QA  BreakpointsForDimension3=[5, 7]  Table=admireDB.aerodata_sym.CNEQD.newTable  ExtrapMethod=Clip  InternalRulePriority=Speed  RndMeth=Simplest  InputSameDT=on
      settings: InputPortMap=u0,u1
  Product : Product
  Cnqd : Outport
  wires:
  CNEQD_QA_M/1 -> Product/2
  Product/1 -> Cnqd/1
  in_bus/1 -> Bus Selector/1  "in_bus"
  Bus Selector/1 -> Product/1  "<qd>"
  Bus Selector/3 -> CNEQD_QA_M/2  "<qacorr>"
  Bus Selector/2 -> CNEQD_QA_M/1  "<mach_nd>"

== system kamerol/Aerodynamics/NormalForceCoefficient/MachRegion2/eoeff ==
  AeroIn_Bus : Inport
  Abs : Abs
  Bus Selector : BusSelector  OutputSignals=mach_nd,angleOfAttack_deg
  CNDEYODE_ALFA_M : Lookup_n-D  BreakpointsForDimension1=admireDB.aerodata_sym.CNDEYODE.breakpoints.M  BreakpointsForDimension2=admireDB.aerodata_sym.CNDEYODE.breakpoints.ALFA  BreakpointsForDimension3=[5, 7]  Table=admireDB.aerodata_sym.CNDEYODE.newTable  ExtrapMethod=Clip  InternalRulePriority=Speed  RndMeth=Simplest  InputSameDT=on
      settings: InputPortMap=u0,u1
  Constant : Constant
  Sum : Sum  Inputs=-+|
  eoeff : Outport
  eieff : Outport  Port=2
  wires:
  AeroIn_Bus/1 -> Bus Selector/1
  Bus Selector/1 -> CNDEYODE_ALFA_M/1  "<mach_nd>"
  Constant/1 -> Sum/2
  CNDEYODE_ALFA_M/1 -> Sum/1, eoeff/1
  Sum/1 -> eieff/1
  Bus Selector/2 -> Abs/1  "<angleOfAttack_deg>"
  Abs/1 -> CNDEYODE_ALFA_M/2

== system kamerol/Aerodynamics/NormalForceCoefficient/MachRegion3/Cnalfa ==
  in_bus : Inport
  Bus Selector : BusSelector  OutputSignals=AeroIn_Bus.angleOfAttack_deg,AeroIn_Bus.mach_nd,AeroIn_Bus.qacorr
  CNEA_QA_M : Lookup_n-D  BreakpointsForDimension1=admireDB.aerodata_sym.CNEA.breakpoints.M  BreakpointsForDimension2=admireDB.aerodata_sym.CNEA.breakpoints.QA  BreakpointsForDimension3=[5, 7]  Table=admireDB.aerodata_sym.CNEA.newTable  ExtrapMethod=Clip  InternalRulePriority=Speed  RndMeth=Simplest  InputSameDT=on
      settings: InputPortMap=u0,u1
  CNMDEA_ALFA_DE_M : Lookup_n-D  NumberOfTableDimensions=3  BreakpointsForDimension1=admireDB.aerodata_sym.CNMDEA.breakpoints.ALFA  BreakpointsForDimension2=admireDB.aerodata_sym.CNMDEA.breakpoints.DE  BreakpointsForDimension3=admireDB.aerodata_sym.CNMDEA.breakpoints.M  Table=admireDB.aerodata_sym.CNMDEA.newTable  ExtrapMethod=Clip  InternalRulePriority=Speed  RndMeth=Simplest  InputSameDT=on
      settings: InputPortMap=u0,u1,u2
  Constant : Constant  Value=0
  Product : Product
  Cnalfa : Outport
  wires:
  Constant/1 -> CNMDEA_ALFA_DE_M/2
  in_bus/1 -> Bus Selector/1  "in_bus"
  Bus Selector/1 -> CNMDEA_ALFA_DE_M/1  "<angleOfAttack_deg>"
  Bus Selector/3 -> CNEA_QA_M/2  "<qacorr>"
  Bus Selector/2 -> CNMDEA_ALFA_DE_M/3, CNEA_QA_M/1  "<mach_nd>"
  CNEA_QA_M/1 -> Product/2
  CNMDEA_ALFA_DE_M/1 -> Product/1
  Product/1 -> Cnalfa/1

== system kamerol/Aerodynamics/NormalForceCoefficient/MachRegion3/Cnalfad ==
  in_bus : Inport
  Abs : Abs
  Bus Selector : BusSelector  OutputSignals=AeroIn_Bus.mach_nd,AeroIn_Bus.angleOfAttack_deg,AeroIn_Bus.alfad
  CNADAM_ALFA_M : Lookup_n-D  BreakpointsForDimension1=admireDB.aerodata_sym.CNADAM.breakpoints.M  BreakpointsForDimension2=admireDB.aerodata_sym.CNADAM.breakpoints.ALFA  BreakpointsForDimension3=[5, 7]  Table=admireDB.aerodata_sym.CNADAM.newTable  ExtrapMethod=Clip  InternalRulePriority=Speed  RndMeth=Simplest  InputSameDT=on
      settings: InputPortMap=u0,u1
  Product : Product
  Cnalfad : Outport
  wires:
  Bus Selector/3 -> Product/2  "<alfad>"
  CNADAM_ALFA_M/1 -> Product/1
  Bus Selector/2 -> Abs/1  "<angleOfAttack_deg>"
  in_bus/1 -> Bus Selector/1  "in_bus"
  Product/1 -> Cnalfad/1
  Bus Selector/1 -> CNADAM_ALFA_M/1  "<mach_nd>"
  Abs/1 -> CNADAM_ALFA_M/2

== system kamerol/Aerodynamics/NormalForceCoefficient/MachRegion3/Cnbasic ==
  in_bus : Inport
  Bus Selector : BusSelector  OutputSignals=AeroIn_Bus.mach_nd,AeroIn_Bus.qacorr
  CNEZERO_QA_M : Lookup_n-D  BreakpointsForDimension1=admireDB.aerodata_sym.CNEZERO.breakpoints.M  BreakpointsForDimension2=admireDB.aerodata_sym.CNEZERO.breakpoints.QA  BreakpointsForDimension3=[5, 7]  Table=admireDB.aerodata_sym.CNEZERO.newTable  ExtrapMethod=Clip  InternalRulePriority=Speed  RndMeth=Simplest  InputSameDT=on
      settings: InputPortMap=u0,u1
  CNZERO_M : Lookup_n-D  NumberOfTableDimensions=1  BreakpointsForDimension1=admireDB.aerodata_sym.CNZERO.breakpoints.M  BreakpointsForDimension3=[5, 7]  Table=admireDB.aerodata_sym.CNZERO.newTable  ExtrapMethod=Clip  InternalRulePriority=Speed  RndMeth=Simplest  InputSameDT=on
  Sum1 : Sum  Inputs=|++
  Cnbasic : Outport
  wires:
  in_bus/1 -> Bus Selector/1  "in_bus"
  Sum1/1 -> Cnbasic/1
  Bus Selector/1 -> CNZERO_M/1, CNEZERO_QA_M/1  "<mach_nd>"
  Bus Selector/2 -> CNEZERO_QA_M/2  "<qacorr>"
  CNZERO_M/1 -> Sum1/1
  CNEZERO_QA_M/1 -> Sum1/2

== system kamerol/Aerodynamics/NormalForceCoefficient/MachRegion3/Cnbeta ==
  Constant : Constant  Value=0
  Cnbeta : Outport
  wires:
  Constant/1 -> Cnbeta/1

== system kamerol/Aerodynamics/NormalForceCoefficient/MachRegion3/Cncai ==
  in_bus : Inport
  Bus Selector : BusSelector  OutputSignals=AeroIn_Bus.angleOfAttack_deg,AeroIn_Bus.cai
  CNCAI_CAI_ALFA : Lookup_n-D  BreakpointsForDimension1=admireDB.aerodata_sym.CNCAI.breakpoints.ALFA  BreakpointsForDimension2=admireDB.aerodata_sym.CNCAI.breakpoints.CAI  BreakpointsForDimension3=[5, 7]  Table=admireDB.aerodata_sym.CNCAI.newTable  ExtrapMethod=Clip  InternalRulePriority=Speed  RndMeth=Simplest  InputSameDT=on
      settings: InputPortMap=u0,u1
  Cncai : Outport
  wires:
  CNCAI_CAI_ALFA/1 -> Cncai/1
  in_bus/1 -> Bus Selector/1  "in_bus"
  Bus Selector/2 -> CNCAI_CAI_ALFA/2  "<cai>"
  Bus Selector/1 -> CNCAI_CAI_ALFA/1  "<angleOfAttack_deg>"

== system kamerol/Aerodynamics/NormalForceCoefficient/MachRegion3/Cndedn ==
  Constant : Constant  Value=0
  Cndedn : Outport
  wires:
  Constant/1 -> Cndedn/1

== system kamerol/Aerodynamics/NormalForceCoefficient/MachRegion3/Cndei ==
  in_bus : Inport
  Bus Selector : BusSelector  OutputSignals=AeroIn_Bus.angleOfAttack_deg,AeroIn_Bus.dEI,AeroIn_Bus.mach_nd,eieff,AeroIn_Bus.qacorr
  CNEDEI_QA_M : Lookup_n-D  BreakpointsForDimension1=admireDB.aerodata_sym.CNEDEI.breakpoints.M  BreakpointsForDimension2=admireDB.aerodata_sym.CNEDEI.breakpoints.QA  BreakpointsForDimension3=[5, 7]  Table=admireDB.aerodata_sym.CNEDEI.newTable  ExtrapMethod=Clip  InternalRulePriority=Speed  RndMeth=Simplest  InputSameDT=on
      settings: InputPortMap=u0,u1
  Product : Product
  Subsystem : Subsystem
  Cndei : Outport
  wires:
  Product/1 -> Cndei/1
  Subsystem/1(Out1) -> Product/1
  Bus Selector/1 -> Subsystem/1(<angleOfAttack_deg>)  "<angleOfAttack_deg>"
  Bus Selector/2 -> Subsystem/2(<dEI>)  "<dEI>"
  Bus Selector/4 -> Subsystem/4(<eieff>)  "<eieff>"
  in_bus/1 -> Bus Selector/1  "in_bus"
  Bus Selector/5 -> CNEDEI_QA_M/2  "<qacorr>"
  Bus Selector/3 -> Subsystem/3(<mach_nd>), CNEDEI_QA_M/1  "<mach_nd>"
  CNEDEI_QA_M/1 -> Product/2

== system kamerol/Aerodynamics/NormalForceCoefficient/MachRegion3/Cndey ==
  in_bus : Inport
  Bus Selector : BusSelector  OutputSignals=AeroIn_Bus.angleOfAttack_deg,AeroIn_Bus.dEY,AeroIn_Bus.mach_nd,eieff,AeroIn_Bus.qacorr
  CNEDEY_QA_M : Lookup_n-D  BreakpointsForDimension1=admireDB.aerodata_sym.CNEDEY.breakpoints.M  BreakpointsForDimension2=admireDB.aerodata_sym.CNEDEY.breakpoints.QA  BreakpointsForDimension3=[5, 7]  Table=admireDB.aerodata_sym.CNEDEY.newTable  ExtrapMethod=Clip  InternalRulePriority=Speed  RndMeth=Simplest  InputSameDT=on
      settings: InputPortMap=u0,u1
  Product : Product
  Subsystem : Subsystem
  Cndey : Outport
  wires:
  CNEDEY_QA_M/1 -> Product/2
  Bus Selector/3 -> Subsystem/3(<mach_nd>), CNEDEY_QA_M/1  "<mach_nd>"
  Bus Selector/5 -> CNEDEY_QA_M/2  "<qacorr>"
  in_bus/1 -> Bus Selector/1  "in_bus"
  Bus Selector/4 -> Subsystem/4(<eieff>)  "<eieff>"
  Bus Selector/2 -> Subsystem/2(<dEI>)  "<dEY>"
  Bus Selector/1 -> Subsystem/1(<angleOfAttack_deg>)  "<angleOfAttack_deg>"
  Subsystem/1(Out1) -> Product/1
  Product/1 -> Cndey/1

== system kamerol/Aerodynamics/NormalForceCoefficient/MachRegion3/Cndle ==
  in_bus : Inport
  Bus Selector : BusSelector  OutputSignals=AeroIn_Bus.angleOfAttack_deg,AeroIn_Bus.mach_nd,AeroIn_Bus.lef_deg
  CNMDLEA_ALFA_DLE_M : Lookup_n-D  NumberOfTableDimensions=3  BreakpointsForDimension1=admireDB.aerodata_sym.CNMDLEA.breakpoints.ALFA  BreakpointsForDimension2=admireDB.aerodata_sym.CNMDLEA.breakpoints.DLE  BreakpointsForDimension3=admireDB.aerodata_sym.CNMDLEA.breakpoints.M  Table=admireDB.aerodata_sym.CNMDLEA.newTable  ExtrapMethod=Clip  InternalRulePriority=Speed  RndMeth=Simplest  InputSameDT=on
      settings: InputPortMap=u0,u1,u2
  Cndle : Outport
  wires:
  CNMDLEA_ALFA_DLE_M/1 -> Cndle/1
  Bus Selector/3 -> CNMDLEA_ALFA_DLE_M/3  "<lef_deg>"
  Bus Selector/2 -> CNMDLEA_ALFA_DLE_M/2  "<mach_nd>"
  Bus Selector/1 -> CNMDLEA_ALFA_DLE_M/1  "<angleOfAttack_deg>"
  in_bus/1 -> Bus Selector/1  "in_bus"
